simulink subsystem "navBusCreator"  (R2026a)
settings: Solver=VariableStepAuto
settings Model: Creator=maxhu  LastModifiedBy=maxhu

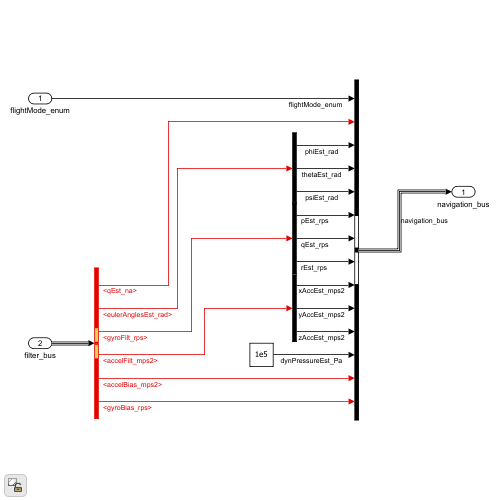
[thumbnail: Simulink's stored preview of the top-level diagram]
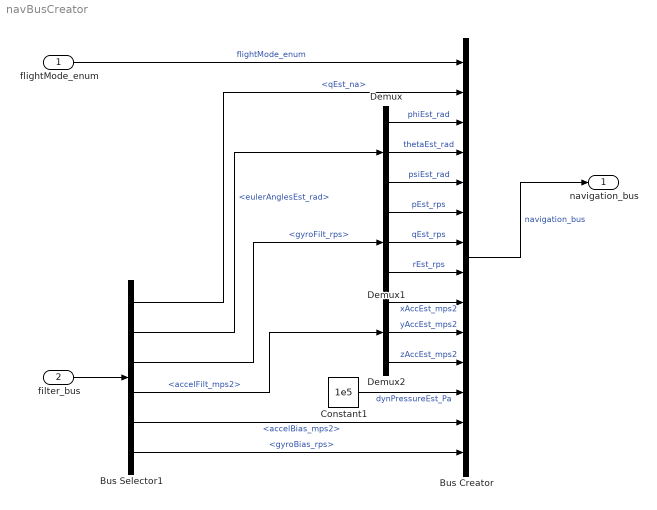
== system navBusCreator ==
  flightMode_enum : Inport
  filter_bus : Inport  Port=2
  Bus Creator : BusCreator  Inputs=14
  Bus Selector1 : BusSelector  OutputSignals=qEst_na,eulerAnglesEst_rad,gyroFilt_rps,accelFilt_mps2,accelBias_mps2,gyroBias_rps
  Constant1 : Constant  Value=1e5
  Demux : Demux  Outputs=3
  Demux1 : Demux  Outputs=3
  Demux2 : Demux  Outputs=3
  navigation_bus : Outport
  wires:
  Demux/2 -> Bus Creator/4  "thetaEst_rad"
  Demux/1 -> Bus Creator/3  "phiEst_rad"
  Demux1/3 -> Bus Creator/8  "rEst_rps"
  Demux/3 -> Bus Creator/5  "psiEst_rad"
  Demux1/1 -> Bus Creator/6  "pEst_rps"
  Constant1/1 -> Bus Creator/12  "dynPressureEst_Pa"
  Demux1/2 -> Bus Creator/7  "qEst_rps"
  Bus Creator/1 -> navigation_bus/1  "navigation_bus"
  Bus Selector1/2 -> Demux/1  "<eulerAnglesEst_rad>"
  flightMode_enum/1 -> Bus Creator/1  "flightMode_enum"
  filter_bus/1 -> Bus Selector1/1
  Bus Selector1/1 -> Bus Creator/2  "<qEst_na>"
  Demux2/1 -> Bus Creator/9  "xAccEst_mps2"
  Demux2/2 -> Bus Creator/10  "yAccEst_mps2"
  Demux2/3 -> Bus Creator/11  "zAccEst_mps2"
  Bus Selector1/5 -> Bus Creator/13  "<accelBias_mps2>"
  Bus Selector1/6 -> Bus Creator/14  "<gyroBias_rps>"
  Bus Selector1/3 -> Demux1/1  "<gyroFilt_rps>"
  Bus Selector1/4 -> Demux2/1  "<accelFilt_mps2>"
